simulink model "throttlePosSend"  (R2019b)
settings: Solver=VariableStepAuto  StartTime=550  StopTime=700  RelTol=1e-3
undefined symbols (not defined in the file or in its folder): canChannel
libraries: canlib x2, simulink x1, canmsglib x1
settings Model: EnablePacing=on  Creator=Nick  LastModifiedBy=Nick

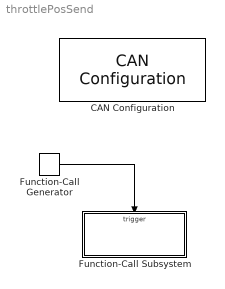
== system throttlePosSend ==
  CAN Configuration : canlib/CAN Configuration  BlockHandle=15256.0002  Device=Vector VN5610 1 (Channel 4)  DeviceMenu=Vector VN5610 1 (Channel 4)  ObjConstructor=canChannel('Vector', 'VN5610 1', 4)  BusSpeed=1000000  EnableBitParameters=off  SJW=2  TSEG1=5  TSEG2=2  NSamples=1  AckMode=Normal
      settings: SourceProductName=Vehicle Network Toolbox  SourceProductBaseCode=VN
  Function-Call Generator : simulink/Ports & Subsystems/Function-Call Generator  sample_time=.001  numberOfIterations=1
  Function-Call Subsystem : Subsystem  TreatAsAtomicUnit=on
  wires:
  Function-Call Generator/1 -> Function-Call Subsystem/Trigger

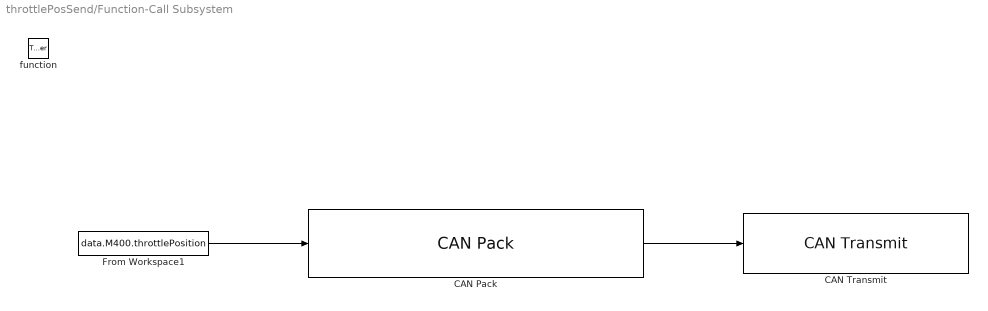
== system throttlePosSend/Function-Call Subsystem ==
  function : TriggerPort  TriggerType=function-call  VariantControl=Variant
  CAN Pack : canmsglib/CAN Pack  CANdbFile=C:\Git\ETC-Development\DBCs\etc_benchTest.dbc  MsgList=VBOX_cmd1  MsgName=VBOX_cmd1  MsgIDType=Standard (11-bit identifier)  MsgIdentifier=500  MsgLength=2  Remote=off  ApplyMinMax=off  BusOutput=off  SignalInfo={'VBOX_throttleCmd','0','16','LE','signed','Standard','0','0.01','0','-327.68','327.67'}
      settings: SourceProductName=Vehicle Network Toolbox  SourceProductBaseCode=VN  DataFormat=CANdb specified signals
  CAN Transmit : canlib/CAN Transmit  BlockHandle=15261.0002  Device=Vector VN5610 1 (Channel 4)  DeviceMenu=Vector VN5610 1 (Channel 4)  ObjConstructor=canChannel('Vector', 'VN5610 1', 4)  EnablePeriodicTransmit=off  MessagePeriod=1.000
      settings: SourceProductName=Vehicle Network Toolbox  SourceProductBaseCode=VN
  From Workspace1 : FromWorkspace  VariableName=data.M400.throttlePosition
  wires:
  CAN Pack/1 -> CAN Transmit/1
  From Workspace1/1 -> CAN Pack/1
